simulink model "quadruped_sim"  (R2023b)
settings: Solver=VariableStepAuto  StartTime=0.0  StopTime=1  RelTol=1e-3
values from neighbouring files (symbols this model uses):
  m = 12    [mpc.m]    (also in mpc_mohsen.m; mpc_simulink.m; qp_simulink.m)
  N = 4    [gait_testing.m]    (also in locoController.m = 10; locoController_obstacle.m = 10; locoController_stairs.m = 10; mpc.m = 10)
  X = [zeros(3, 1); zeros(3,1); zeros(3,1); zeros(3, 1)]    [mpc_testing.m]    (also in testing_mpc.m = [-0.02; 0; 0.25; zeros(3, 1); zeros(3, 1); zeros(3, 1)])
undefined symbols (not defined in the file or in its folder): Y, Z
libraries: sm_lib x173, nesl_utility x42
(part 4 of 4)

== system quadruped_sim/a1_robot/imu_link ==
  Inertia : sm_lib/Body Elements/Inertia  InertiaType=Custom  Mass=0.001  MassUnits=kg  CenterOfMass=[0, 0, 0]  CenterOfMassUnits=m  MomentsOfInertia=[0.0001, 0.0001, 0.0001]  MomentsOfInertiaUnits=kg*m^2  ProductsOfInertia=[0, 0, 0]  ProductsOfInertiaUnits=kg*m^2  GraphicType=None  MarkerShape=Inertia  MarkerSize=20  GraphicVisPropType=SimpleVisualProperties  GraphicDiffuseColor=[0.5 0.5 0.5]  GraphicSpecularColor=[0.5 0.5 0.5 1.0]  GraphicAmbientColor=[0.15 0.15 0.15 1.0]  GraphicEmissiveColor=[0.0 0.0 0.0 1.0]  GraphicShininess=75  GraphicOpacity=1.0
  InertiaOriginTransform : sm_lib/Frames and Transforms/Rigid Transform  TranslationMethod=Cartesian  TranslationStandardOffset=0  TranslationStandardOffsetUnits=m  TranslationStandardAxis=+Z  TranslationCartesianOffset=[0, 0, 0]  TranslationCartesianOffsetUnits=m  TranslationROffset=0  TranslationROffsetUnits=m  TranslationZOffset=0  TranslationZOffsetUnits=m  TranslationThetaOffset=0  TranslationThetaOffsetUnits=deg  RotationMethod=RotationSequence  RotationAngleUnits=deg  RotationStandardAxis=+Z  RotationAngle=0.0  RotationArbitraryAxis=[0 0 1]  FollAlignAxisA=+X  BaseAlignAxisA=+Y  FollAlignAxisB=+Y  BaseAlignAxisB=+Z  RotationSequenceAxes=BaseAxes  RotationSequence=XYZ  RotationSequenceAngles=[0, 0, 0]  RotationSequenceAnglesUnits=rad  RotationMatrix=[1 0 0; 0 1 0; 0 0 1]  Quaternion=[1 0 0 0]
  ReferenceFrame : sm_lib/Frames and Transforms/Reference Frame
  Visual : sm_lib/Body Elements/Brick Solid  GraphicAmbientColor=[0.15 0.15 0.15 1.0]  BasedOnType=Density  BrickDimensions=[0.001, 0.001, 0.001]  BrickDimensionsUnits=m  CenterOfMass=[0, 0, 0]  CenterOfMassUnits=m  GraphicDiffuseColor=[0.8, 0, 0]  Density=1000  DensityUnits=kg/m^3  DoExposeReferenceFrame=on  GraphicEmissiveColor=[0.0 0.0 0.0 1.0]  ExportEntireGeometry=off  SerializedFrames=<Frames/>  MarkerShape=Sphere  MarkerSize=10  GraphicType=FromGeometry  InertiaType=Custom  Mass=0  MassUnits=kg  MomentsOfInertia=[0, 0, 0]  MomentsOfInertiaUnits=kg*m^2  GraphicOpacity=1  ProductsOfInertia=[0, 0, 0]  ProductsOfInertiaUnits=kg*m^2  GraphicShininess=75  GraphicSpecularColor=[0.5 0.5 0.5 1.0]  GraphicVisPropType=SimpleVisualProperties
  VisualOriginTransform : sm_lib/Frames and Transforms/Rigid Transform  TranslationMethod=Cartesian  TranslationStandardOffset=0  TranslationStandardOffsetUnits=m  TranslationStandardAxis=+Z  TranslationCartesianOffset=[0, 0, 0]  TranslationCartesianOffsetUnits=m  TranslationROffset=0  TranslationROffsetUnits=m  TranslationZOffset=0  TranslationZOffsetUnits=m  TranslationThetaOffset=0  TranslationThetaOffsetUnits=deg  RotationMethod=RotationSequence  RotationAngleUnits=deg  RotationStandardAxis=+Z  RotationAngle=0.0  RotationArbitraryAxis=[0 0 1]  FollAlignAxisA=+X  BaseAlignAxisA=+Y  FollAlignAxisB=+Y  BaseAlignAxisB=+Z  RotationSequenceAxes=BaseAxes  RotationSequence=XYZ  RotationSequenceAngles=[0, 0, 0]  RotationSequenceAnglesUnits=rad  RotationMatrix=[1 0 0; 0 1 0; 0 0 1]  Quaternion=[1 0 0 0]
  F : PMIOPort  Side=Left
  connections:
  Inertia/RConn1 -- InertiaOriginTransform/RConn1
  ReferenceFrame/RConn1 -- InertiaOriginTransform/LConn1 -- VisualOriginTransform/LConn1 -- F/RConn1
  Visual/RConn1 -- VisualOriginTransform/RConn1

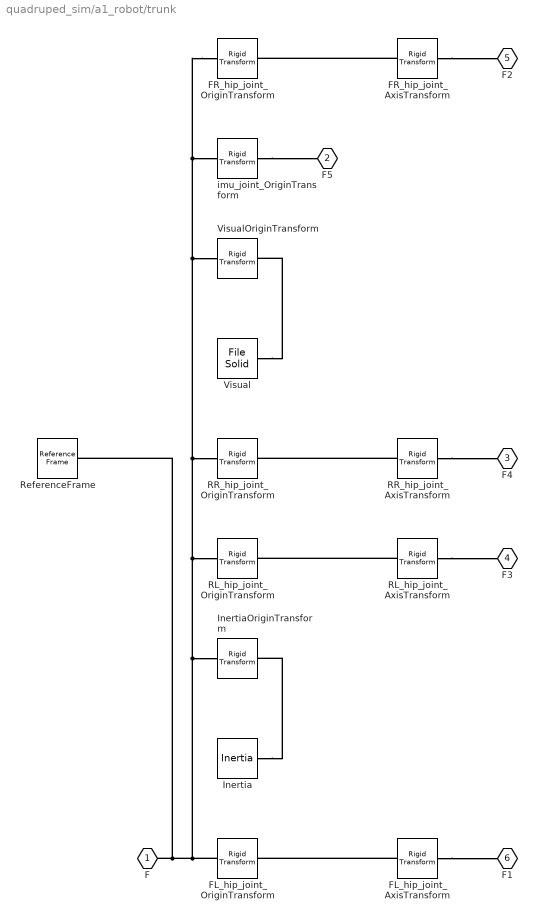
== system quadruped_sim/a1_robot/trunk ==
  FL_hip_joint_AxisTransform : sm_lib/Frames and Transforms/Rigid Transform  TranslationMethod=Cartesian  TranslationStandardOffset=0  TranslationStandardOffsetUnits=m  TranslationStandardAxis=+Z  TranslationCartesianOffset=[0, 0, 0]  TranslationCartesianOffsetUnits=m  TranslationROffset=0  TranslationROffsetUnits=m  TranslationZOffset=0  TranslationZOffsetUnits=m  TranslationThetaOffset=0  TranslationThetaOffsetUnits=deg  RotationMethod=ArbitraryAxis  RotationAngleUnits=rad  RotationStandardAxis=+Z  RotationAngle=1.570796326794897  RotationArbitraryAxis=[-0, 1, 0]  FollAlignAxisA=+X  BaseAlignAxisA=+Y  FollAlignAxisB=+Y  BaseAlignAxisB=+Z  RotationSequenceAxes=FollowerAxes  RotationSequence=XYX  RotationSequenceAngles=[0 0 0]  RotationSequenceAnglesUnits=deg  RotationMatrix=[1 0 0; 0 1 0; 0 0 1]  Quaternion=[1 0 0 0]
  FL_hip_joint_OriginTransform : sm_lib/Frames and Transforms/Rigid Transform  TranslationMethod=Cartesian  TranslationStandardOffset=0  TranslationStandardOffsetUnits=m  TranslationStandardAxis=+Z  TranslationCartesianOffset=[0.1805, 0.047, 0]  TranslationCartesianOffsetUnits=m  TranslationROffset=0  TranslationROffsetUnits=m  TranslationZOffset=0  TranslationZOffsetUnits=m  TranslationThetaOffset=0  TranslationThetaOffsetUnits=deg  RotationMethod=RotationSequence  RotationAngleUnits=deg  RotationStandardAxis=+Z  RotationAngle=0.0  RotationArbitraryAxis=[0 0 1]  FollAlignAxisA=+X  BaseAlignAxisA=+Y  FollAlignAxisB=+Y  BaseAlignAxisB=+Z  RotationSequenceAxes=BaseAxes  RotationSequence=XYZ  RotationSequenceAngles=[0, 0, 0]  RotationSequenceAnglesUnits=rad  RotationMatrix=[1 0 0; 0 1 0; 0 0 1]  Quaternion=[1 0 0 0]
  FR_hip_joint_AxisTransform : sm_lib/Frames and Transforms/Rigid Transform  TranslationMethod=Cartesian  TranslationStandardOffset=0  TranslationStandardOffsetUnits=m  TranslationStandardAxis=+Z  TranslationCartesianOffset=[0, 0, 0]  TranslationCartesianOffsetUnits=m  TranslationROffset=0  TranslationROffsetUnits=m  TranslationZOffset=0  TranslationZOffsetUnits=m  TranslationThetaOffset=0  TranslationThetaOffsetUnits=deg  RotationMethod=ArbitraryAxis  RotationAngleUnits=rad  RotationStandardAxis=+Z  RotationAngle=1.570796326794897  RotationArbitraryAxis=[-0, 1, 0]  FollAlignAxisA=+X  BaseAlignAxisA=+Y  FollAlignAxisB=+Y  BaseAlignAxisB=+Z  RotationSequenceAxes=FollowerAxes  RotationSequence=XYX  RotationSequenceAngles=[0 0 0]  RotationSequenceAnglesUnits=deg  RotationMatrix=[1 0 0; 0 1 0; 0 0 1]  Quaternion=[1 0 0 0]
  FR_hip_joint_OriginTransform : sm_lib/Frames and Transforms/Rigid Transform  TranslationMethod=Cartesian  TranslationStandardOffset=0  TranslationStandardOffsetUnits=m  TranslationStandardAxis=+Z  TranslationCartesianOffset=[0.1805, -0.047, 0]  TranslationCartesianOffsetUnits=m  TranslationROffset=0  TranslationROffsetUnits=m  TranslationZOffset=0  TranslationZOffsetUnits=m  TranslationThetaOffset=0  TranslationThetaOffsetUnits=deg  RotationMethod=RotationSequence  RotationAngleUnits=deg  RotationStandardAxis=+Z  RotationAngle=0.0  RotationArbitraryAxis=[0 0 1]  FollAlignAxisA=+X  BaseAlignAxisA=+Y  FollAlignAxisB=+Y  BaseAlignAxisB=+Z  RotationSequenceAxes=BaseAxes  RotationSequence=XYZ  RotationSequenceAngles=[0, 0, 0]  RotationSequenceAnglesUnits=rad  RotationMatrix=[1 0 0; 0 1 0; 0 0 1]  Quaternion=[1 0 0 0]
  Inertia : sm_lib/Body Elements/Inertia  InertiaType=Custom  Mass=6  MassUnits=kg  CenterOfMass=[0, 0, 0]  CenterOfMassUnits=m  MomentsOfInertia=[0.0158533, 0.0377999, 0.0456542]  MomentsOfInertiaUnits=kg*m^2  ProductsOfInertia=[-2.75e-05, -6.109999999999999e-05, -3.66e-05]  ProductsOfInertiaUnits=kg*m^2  GraphicType=None  MarkerShape=Inertia  MarkerSize=20  GraphicVisPropType=SimpleVisualProperties  GraphicDiffuseColor=[0.5 0.5 0.5]  GraphicSpecularColor=[0.5 0.5 0.5 1.0]  GraphicAmbientColor=[0.15 0.15 0.15 1.0]  GraphicEmissiveColor=[0.0 0.0 0.0 1.0]  GraphicShininess=75  GraphicOpacity=1.0
  InertiaOriginTransform : sm_lib/Frames and Transforms/Rigid Transform  TranslationMethod=Cartesian  TranslationStandardOffset=0  TranslationStandardOffsetUnits=m  TranslationStandardAxis=+Z  TranslationCartesianOffset=[0, 0.0041, -0.0005]  TranslationCartesianOffsetUnits=m  TranslationROffset=0  TranslationROffsetUnits=m  TranslationZOffset=0  TranslationZOffsetUnits=m  TranslationThetaOffset=0  TranslationThetaOffsetUnits=deg  RotationMethod=RotationSequence  RotationAngleUnits=deg  RotationStandardAxis=+Z  RotationAngle=0.0  RotationArbitraryAxis=[0 0 1]  FollAlignAxisA=+X  BaseAlignAxisA=+Y  FollAlignAxisB=+Y  BaseAlignAxisB=+Z  RotationSequenceAxes=BaseAxes  RotationSequence=XYZ  RotationSequenceAngles=[0, 0, 0]  RotationSequenceAnglesUnits=rad  RotationMatrix=[1 0 0; 0 1 0; 0 0 1]  Quaternion=[1 0 0 0]
  RL_hip_joint_AxisTransform : sm_lib/Frames and Transforms/Rigid Transform  TranslationMethod=Cartesian  TranslationStandardOffset=0  TranslationStandardOffsetUnits=m  TranslationStandardAxis=+Z  TranslationCartesianOffset=[0, 0, 0]  TranslationCartesianOffsetUnits=m  TranslationROffset=0  TranslationROffsetUnits=m  TranslationZOffset=0  TranslationZOffsetUnits=m  TranslationThetaOffset=0  TranslationThetaOffsetUnits=deg  RotationMethod=ArbitraryAxis  RotationAngleUnits=rad  RotationStandardAxis=+Z  RotationAngle=1.570796326794897  RotationArbitraryAxis=[-0, 1, 0]  FollAlignAxisA=+X  BaseAlignAxisA=+Y  FollAlignAxisB=+Y  BaseAlignAxisB=+Z  RotationSequenceAxes=FollowerAxes  RotationSequence=XYX  RotationSequenceAngles=[0 0 0]  RotationSequenceAnglesUnits=deg  RotationMatrix=[1 0 0; 0 1 0; 0 0 1]  Quaternion=[1 0 0 0]
  RL_hip_joint_OriginTransform : sm_lib/Frames and Transforms/Rigid Transform  TranslationMethod=Cartesian  TranslationStandardOffset=0  TranslationStandardOffsetUnits=m  TranslationStandardAxis=+Z  TranslationCartesianOffset=[-0.1805, 0.047, 0]  TranslationCartesianOffsetUnits=m  TranslationROffset=0  TranslationROffsetUnits=m  TranslationZOffset=0  TranslationZOffsetUnits=m  TranslationThetaOffset=0  TranslationThetaOffsetUnits=deg  RotationMethod=RotationSequence  RotationAngleUnits=deg  RotationStandardAxis=+Z  RotationAngle=0.0  RotationArbitraryAxis=[0 0 1]  FollAlignAxisA=+X  BaseAlignAxisA=+Y  FollAlignAxisB=+Y  BaseAlignAxisB=+Z  RotationSequenceAxes=BaseAxes  RotationSequence=XYZ  RotationSequenceAngles=[0, 0, 0]  RotationSequenceAnglesUnits=rad  RotationMatrix=[1 0 0; 0 1 0; 0 0 1]  Quaternion=[1 0 0 0]
  RR_hip_joint_AxisTransform : sm_lib/Frames and Transforms/Rigid Transform  TranslationMethod=Cartesian  TranslationStandardOffset=0  TranslationStandardOffsetUnits=m  TranslationStandardAxis=+Z  TranslationCartesianOffset=[0, 0, 0]  TranslationCartesianOffsetUnits=m  TranslationROffset=0  TranslationROffsetUnits=m  TranslationZOffset=0  TranslationZOffsetUnits=m  TranslationThetaOffset=0  TranslationThetaOffsetUnits=deg  RotationMethod=ArbitraryAxis  RotationAngleUnits=rad  RotationStandardAxis=+Z  RotationAngle=1.570796326794897  RotationArbitraryAxis=[-0, 1, 0]  FollAlignAxisA=+X  BaseAlignAxisA=+Y  FollAlignAxisB=+Y  BaseAlignAxisB=+Z  RotationSequenceAxes=FollowerAxes  RotationSequence=XYX  RotationSequenceAngles=[0 0 0]  RotationSequenceAnglesUnits=deg  RotationMatrix=[1 0 0; 0 1 0; 0 0 1]  Quaternion=[1 0 0 0]
  RR_hip_joint_OriginTransform : sm_lib/Frames and Transforms/Rigid Transform  TranslationMethod=Cartesian  TranslationStandardOffset=0  TranslationStandardOffsetUnits=m  TranslationStandardAxis=+Z  TranslationCartesianOffset=[-0.1805, -0.047, 0]  TranslationCartesianOffsetUnits=m  TranslationROffset=0  TranslationROffsetUnits=m  TranslationZOffset=0  TranslationZOffsetUnits=m  TranslationThetaOffset=0  TranslationThetaOffsetUnits=deg  RotationMethod=RotationSequence  RotationAngleUnits=deg  RotationStandardAxis=+Z  RotationAngle=0.0  RotationArbitraryAxis=[0 0 1]  FollAlignAxisA=+X  BaseAlignAxisA=+Y  FollAlignAxisB=+Y  BaseAlignAxisB=+Z  RotationSequenceAxes=BaseAxes  RotationSequence=XYZ  RotationSequenceAngles=[0, 0, 0]  RotationSequenceAnglesUnits=rad  RotationMatrix=[1 0 0; 0 1 0; 0 0 1]  Quaternion=[1 0 0 0]
  ReferenceFrame : sm_lib/Frames and Transforms/Reference Frame
  Visual : sm_lib/Body Elements/File Solid  ExtGeomFileName=a1_description/meshes/trunk.stl  UnitType=Custom  ExtGeomFileUnits=m  StepReaderType=HEX  ExportConvexHullGeometry=off  InertiaType=Custom  Mass=0  MassUnits=kg  CenterOfMass=[0, 0, 0]  CenterOfMassUnits=m  MomentsOfInertia=[0, 0, 0]  MomentsOfInertiaUnits=kg*m^2  ProductsOfInertia=[0, 0, 0]  ProductsOfInertiaUnits=kg*m^2  BasedOnType=DensityFromFile  Density=1000  DensityUnits=kg/m^3  DoExposeReferenceFrame=on  SerializedFrames=<Frames/>  GraphicType=FromGeometry  MarkerShape=Sphere  MarkerSize=10  GraphicVisPropType=SimpleVisualProperties  GraphicDiffuseColor=[1, 0.423529411765, 0.0392156862745]  GraphicSpecularColor=[0.5 0.5 0.5 1.0]  GraphicAmbientColor=[0.15 0.15 0.15 1.0]  GraphicEmissiveColor=[0.0 0.0 0.0 1.0]  GraphicShininess=75  GraphicOpacity=1
  VisualOriginTransform : sm_lib/Frames and Transforms/Rigid Transform  TranslationMethod=Cartesian  TranslationStandardOffset=0  TranslationStandardOffsetUnits=m  TranslationStandardAxis=+Z  TranslationCartesianOffset=[0, 0, 0]  TranslationCartesianOffsetUnits=m  TranslationROffset=0  TranslationROffsetUnits=m  TranslationZOffset=0  TranslationZOffsetUnits=m  TranslationThetaOffset=0  TranslationThetaOffsetUnits=deg  RotationMethod=RotationSequence  RotationAngleUnits=deg  RotationStandardAxis=+Z  RotationAngle=0.0  RotationArbitraryAxis=[0 0 1]  FollAlignAxisA=+X  BaseAlignAxisA=+Y  FollAlignAxisB=+Y  BaseAlignAxisB=+Z  RotationSequenceAxes=BaseAxes  RotationSequence=XYZ  RotationSequenceAngles=[0, 0, 0]  RotationSequenceAnglesUnits=rad  RotationMatrix=[1 0 0; 0 1 0; 0 0 1]  Quaternion=[1 0 0 0]
  imu_joint_OriginTransform : sm_lib/Frames and Transforms/Rigid Transform  TranslationMethod=Cartesian  TranslationStandardOffset=0  TranslationStandardOffsetUnits=m  TranslationStandardAxis=+Z  TranslationCartesianOffset=[0, 0, 0]  TranslationCartesianOffsetUnits=m  TranslationROffset=0  TranslationROffsetUnits=m  TranslationZOffset=0  TranslationZOffsetUnits=m  TranslationThetaOffset=0  TranslationThetaOffsetUnits=deg  RotationMethod=RotationSequence  RotationAngleUnits=deg  RotationStandardAxis=+Z  RotationAngle=0.0  RotationArbitraryAxis=[0 0 1]  FollAlignAxisA=+X  BaseAlignAxisA=+Y  FollAlignAxisB=+Y  BaseAlignAxisB=+Z  RotationSequenceAxes=BaseAxes  RotationSequence=XYZ  RotationSequenceAngles=[0, 0, 0]  RotationSequenceAnglesUnits=rad  RotationMatrix=[1 0 0; 0 1 0; 0 0 1]  Quaternion=[1 0 0 0]
  F : PMIOPort  Side=Left
  F5 : PMIOPort  Port=2  Side=Right
  F4 : PMIOPort  Port=3  Side=Right
  F3 : PMIOPort  Port=4  Side=Right
  F2 : PMIOPort  Port=5  Side=Right
  F1 : PMIOPort  Port=6  Side=Right
  connections:
  FL_hip_joint_AxisTransform/RConn1 -- F1/RConn1
  FL_hip_joint_AxisTransform/LConn1 -- FL_hip_joint_OriginTransform/RConn1
  FR_hip_joint_AxisTransform/RConn1 -- F2/RConn1
  FR_hip_joint_AxisTransform/LConn1 -- FR_hip_joint_OriginTransform/RConn1
  Inertia/RConn1 -- InertiaOriginTransform/RConn1
  RL_hip_joint_AxisTransform/RConn1 -- F3/RConn1
  RL_hip_joint_AxisTransform/LConn1 -- RL_hip_joint_OriginTransform/RConn1
  RR_hip_joint_AxisTransform/RConn1 -- F4/RConn1
  RR_hip_joint_AxisTransform/LConn1 -- RR_hip_joint_OriginTransform/RConn1
  FR_hip_joint_OriginTransform/LConn1 -- FL_hip_joint_OriginTransform/LConn1 -- ReferenceFrame/RConn1 -- F/RConn1 -- InertiaOriginTransform/LConn1 -- RL_hip_joint_OriginTransform/LConn1 -- RR_hip_joint_OriginTransform/LConn1 -- VisualOriginTransform/LConn1 -- imu_joint_OriginTransform/LConn1
  Visual/RConn1 -- VisualOriginTransform/RConn1
  imu_joint_OriginTransform/RConn1 -- F5/RConn1

== matlab function quadruped_sim/Standing Controller ==
  data: t input; qDes output
function qDes = stand(t)
% qDefault = [0.26; 1.25; -2.7; -0.26; 1.25; -2.7; 0.26; 1.25; -2.7; -0.26; 1.25; -2.7;];
qDefault = [0; 1.25; -2.7; 0; 1.25; -2.7; 0; 1.25; -2.7; 0; 1.25; -2.7;];
qStand = [0; 0.9; -1.7; 0; 0.9; -1.7; 0; 0.9; -1.8; 0; 0.9; -1.7];

if t > 1
    qDes = qStand;
else 
    qDes = qDefault;
end

%{
LR Initial State Target
	Thigh: 1.25
	Calf: -2.7
	Hip: 0.26

Desired (might be old though)
	Hip: 0
	Thigh: 0.2
    Calf: -0.2

%}

== matlab function quadruped_sim/jointPD ==
  data: qDes input; u output; q input; dqDes input; dq input
function u = jointPD(qDes, q, dqDes, dq)
% FL (H, T, C)
% FR (...), RL (...), RF (...)

%         kp_hip = 10;
%         kp_thigh = 10;
%         kp_calf = 10;
%         kd_hip = 1;
%         kd_thigh = 1;
%         kd_calf = 1;
    kp = 60;
    kd = 10;

    u = kp .* (qDes - q) + kd .* (dqDes - dq); 
end

== matlab function quadruped_sim/MATLAB Function1 ==
  data: X input; grf_forces output; pf input
function grf_forces = mpc(X, pf) 
    Xd = [0; 0; 0.3; zeros(3,1); zeros(3,1); zeros(3,1)];
    P = X(1:3);
    ypr = X(4:6);
    X_bard = [Xd; 9.81];
    X_bar = [X; 9.81];
    forces = 4;
    bar_states = 13;
    N = 10;
    dt = 0.03;
    Xmpc_elem = bar_states*N + forces*3*N;


    % Q, R values from HW4 #2(b)
    Q = diag([40, 50, 60, 10, 10, 10, 4, 4, 4, 1, 1, 1, 0]);
    R = 0.00001*eye(forces*3);
    m = 12;
    F_max = 500;
    F_min = 10;
    mu = 0.5;
    I_b = diag([0.0168, 0.0565, 0.064]);
        
    % Foot Contact
    % Would need to update for swing trajectory
%{
ftcontact_prev = params.ftcontact_prev;
    ftcontact_next = gait(1:forces);
    hip_vec = [params.vk, params.vg, params.vi, params.ve];
    for ind = 1:forces
        if ftcontact_prev(ind) == 0 && ftcontact_next(ind) == 1
            r_temp = R*hip_vec(:, ind) + P;
            switch ind
                case 1
                    params.p_f1 = [r_temp(1:2); 0];
                case 2
                    params.p_f2 = [r_temp(1:2); 0];
                case 3
                    params.p_f3 = [r_temp(1:2); 0];
                case 4
                    params.p_f4 = [r_temp(1:2); 0];
            end
        end
    end
%}


    % Cost function parameters
    temp_fQs = [];
    for ind = 1:N
        temp_Qs = [temp_Qs; diag(Q)];
        temp_Rs = [temp_Rs; diag(R)];
        temp_fQs = [temp_fQs; -Q'*X_bard];
    end
    H = diag([temp_Qs; temp_Rs]);
    f = [temp_fQs; zeros(3*forces*N, 1)];

    % Inequality constraints A_iq
    Fiq_mat = [-1, 0, -mu; 1, 0, -mu; 0, -1, -mu; 0, 1, -mu; 0, 0, 1; 0, 0, -1];
    A_iq = [zeros(6*forces*N, bar_states*N), kron(eye(forces*N),Fiq_mat)];


    % Inequality constraints b_iq
    b_iq = [];
    for ind = 1:forces*N
        % alpha = gait(ind);
        alpha = 1;
        b_iq = [b_iq; 0; 0; 0; 0; alpha*F_max; -alpha*F_min];
    end

    % Linearization
    % [Yaw, Pitch, Roll]
    psi = ypr(1);
    theta = ypr(2);
    phi  = ypr(3);

    Rz_T = [cos(psi), sin(psi), 0; -sin(psi), cos(psi), 0; 0, 0, 1];
    I_w = Rz_T'*I_b*Rz_T;

    A_bar = zeros(bar_states);
    A_bar(1:3, 3*2+1:3*3) = eye(3);
    A_bar(3+1:3*2, 3*3+1:3*4) = Rz_T;
    A_bar(3*3, bar_states) = -1;

    % Position of feet in world frame
    r_f1 = pf(1:3) - P;
    r_f2 = pf(4:6) - P;
    r_f3 = pf(7:9) - P;
    r_f4 = pf(10:12) - P;
    r_fs = [r_f1, r_f2, r_f3, r_f4];
    temp_mat = [];
    for ind = 1:forces
        temp_r = r_fs(:, ind);
        temp = [0, -temp_r(3), temp_r(2); temp_r(3), 0, -temp_r(1); -temp_r(2), temp_r(1), 0];
        temp_term = inv(I_w)*temp;
        temp_mat = [temp_mat, temp_term];
    end
    B_bar = [zeros(3*2, 3*forces); [eye(3)/m, eye(3)/m, eye(3)/m, eye(3)/m]; temp_mat; zeros(1, 3*forces)];

    % Discretization
    A_k = A_bar*dt + eye(bar_states);
    B_k = B_bar*dt;

    % MPC Dynamic Constraints
    A_eq = zeros(bar_states, Xmpc_elem - 3*forces*N);
    A_eq(1:bar_states, 1:bar_states) = eye(bar_states);
    A_Xrot = [-A_k, eye(bar_states)];
    A_Xrot = [A_Xrot, zeros(bar_states, bar_states*(N-2))];
    % Shift for each 
    for ind = 1:N-1
        A_eq = [A_eq; A_Xrot];
        A_Xrot = circshift(A_Xrot,bar_states, 2);
    end
    for ind = 1:N
        temp_vec = zeros(Xmpc_elem - 3*forces*N, 1);
        start = 1 + bar_states*(ind - 1);
        temp_vec(start:start+bar_states-1, 1:3*forces) = -B_k; 
        A_eq = [A_eq, temp_vec];
    end

    b_eq = zeros(Xmpc_elem - 3*forces*N, 1);
    b_eq(1:bar_states) = A_k*X_bar;


    X_mpc = quadprog(H, f, A_iq, b_iq, A_eq, b_eq);
    grf_forces = X_mpc(N*bar_states + 1:N*bar_states + 3*forces, 1);
end

== matlab function quadruped_sim/MATLAB Function ==
  data: F input; torques output; Q input; t input; x input; pf output
% Converts force at toe in body frame to resulting joint torques
% Inputs: 
%   F - forces at toe for all 4 legs (12x1). Order is FL,FR,RL,RR
%   q - joints angles for all 4 legs (12x1 in radians). Order is
%   FL,FR,RL,RR
function [torques, pf] = legs_force_to_torque(F, Q, t, x)
    offset_x = 0.1805;
    offset_y = -0.047;
    offset_z = 0.0;
    torques = zeros(12,1);
    % Kinematic parameters
    a1 = 0.045; %m
    a2 = 0.2; %m
    a3 = 0.2; %m
    
    % iterate through legs. Order is FL,FR,RL,RF
    for i = 0:3

        legSign = 1;
        if i == 0 || i == 2
            legSign = -1;
        end
        
        frontBackSign = 1;
        if i == 2 || i == 3
            frontBackSign = -1;
        end

        q = Q(3*i+1:3*i+3);
        f = F(3*i+1:3*i+3);
        %transformation from body frame to hip frame
        % R_B0 = eul2rotm([-pi/2,0,-pi/2]);
        R_B0 = [0 0 1;%for coordinate flipping, before q1 applied
            -1 0 0;
             0 -1 0];
        d_BodyToHip = [offset_x * frontBackSign; offset_y * legSign; offset_z];
        T_B0 = [R_B0,d_BodyToHip;zeros(1,3),1];
        
        %transformation from hip frame to thigh frame
        % R = eul2rotm([pi/2,0,pi/2]); 
        R = [0 0 1;%for coordinate flipping, before q1 applied
            1 0 0;
             0 1 0];
        R_T = [R,[0;0;0];zeros(1,3),1];
        T_01rot = [cos(q(1)) -sin(q(1)) 0 0; sin(q(1)) cos(q(1)) 0 0 ; 0 0 1 0; 0 0 0 1];
        T_01 = T_01rot * R_T; %combine coordinate flip and q1 application
        
        %transformation from thigh to knee frame
        T_12trans = eye(4);
        T_12trans(1:3,4) = [a2; 0; a1*legSign];
        T_12rot = [cos(q(2)) -sin(q(2)) 0 0; sin(q(2)) cos(q(2)) 0 0 ; 0 0 1 0; 0 0 0 1];
        T_12 = T_12rot * T_12trans;
        
        %transformation from knee to toe frame
        T_23trans = eye(4);
        T_23trans(1:3,4) = [a3; 0; 0];
        T_23rot = [cos(q(3)) -sin(q(3)) 0 0; sin(q(3)) cos(q(3)) 0 0 ; 0 0 1 0; 0 0 0 1];
        T_23 = T_23rot * T_23trans;
        
        %compute frame origins (all in body frame)
        P_EE = [0;0;0;1];
        O_0 = T_B0* P_EE;
        O_1 = T_B0* T_01 * P_EE;
        O_2 = T_B0* T_01 * T_12 * P_EE;
        O_3 = T_B0* T_01 * T_12 * T_23 * P_EE;
        
        H_b0 = [eul2rotm(x(4:6)), x(1:3); zeros(1, 3); 1];
        pf = H_b0 * O_3;
        
        %compute joint axes (all in body frame)
        z0 = [1;0;0];
        z1 = [0;-cos(q(1));-sin(q(1))];
        z2 = [0;-cos(q(1));-sin(q(1))];
        
        %compute Jacobian
        J = [cross(z0, O_3(1:3)-O_0(1:3)), ...
            cross(z1, O_3(1:3)-O_1(1:3)), ...
            cross(z2, O_3(1:3)-O_2(1:3))];
        
        torque = J' * f;

        torques(3*i+1:3*i+3) = torque .* [1;-1;1];
    end

    % if  t<1
    %     torques = zeros(12,1);
    % end
end
